simulink model "untitled1"  (Simulink 7.6)
settings: Solver=ode45  StartTime=0.0  StopTime=10.0  RelTol=1e-3
values from neighbouring files (symbols this model uses):
  K = [9.375  -6.25; -8.125  8.75]    [PP2013428.mat]
settings Model: Creator=Administrator  LastModifiedBy=Administrator
settings DebuggingCC: SolverPrmCheckMsg=none

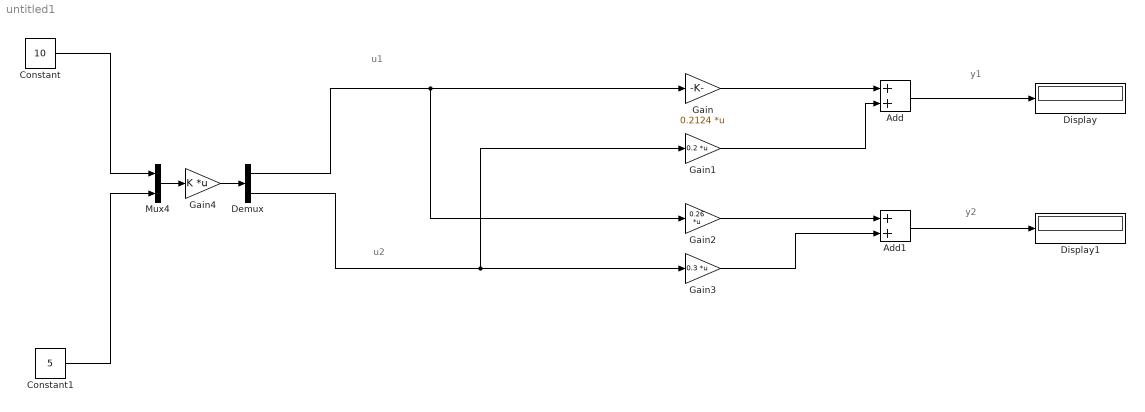
== system untitled1 ==
  note: y1
  note: y2
  note: u1
  note: u2
  Add : Sum
  Add1 : Sum
  Constant : Constant  Value=10
  Constant1 : Constant  Value=5
  Demux : Demux  Outputs=2
  Display : Display
  Display1 : Display
  Gain : Gain  Gain=0.2124  Multiplication=Matrix(K*u)
  Gain1 : Gain  Gain=0.2  Multiplication=Matrix(K*u)
  Gain2 : Gain  Gain=0.26  Multiplication=Matrix(K*u)
  Gain3 : Gain  Gain=0.3  Multiplication=Matrix(K*u)
  Gain4 : Gain  Gain=K  Multiplication=Matrix(K*u)
  Mux4 : Mux  Inputs=2
  wires:
  Demux/1 -> Gain/1, Gain2/1
  Gain/1 -> Add/1
  Gain1/1 -> Add/2
  Add/1 -> Display/1
  Gain2/1 -> Add1/1
  Gain3/1 -> Add1/2
  Add1/1 -> Display1/1
  Demux/2 -> Gain3/1, Gain1/1
  Constant/1 -> Mux4/1
  Constant1/1 -> Mux4/2
  Mux4/1 -> Gain4/1
  Gain4/1 -> Demux/1
